simulink model "ProjectBosch"  (R2024b)
settings: Solver=FixedStepAuto  StartTime=0.0  StopTime=16000  FixedStep=1  RelTol=1e-3
libraries: simulink x5, embmathops x2
settings Model: Creator=user  LastModifiedBy=user

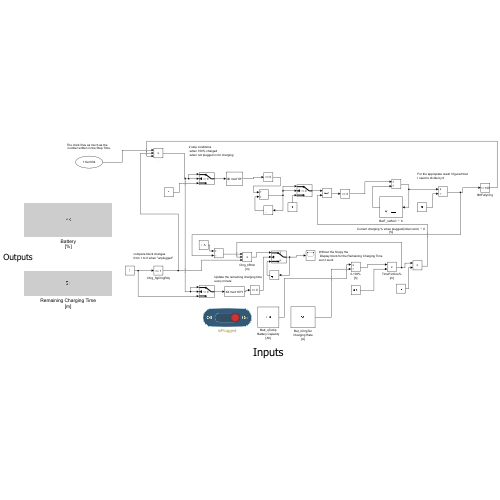
[thumbnail: Simulink's stored preview of the top-level diagram]
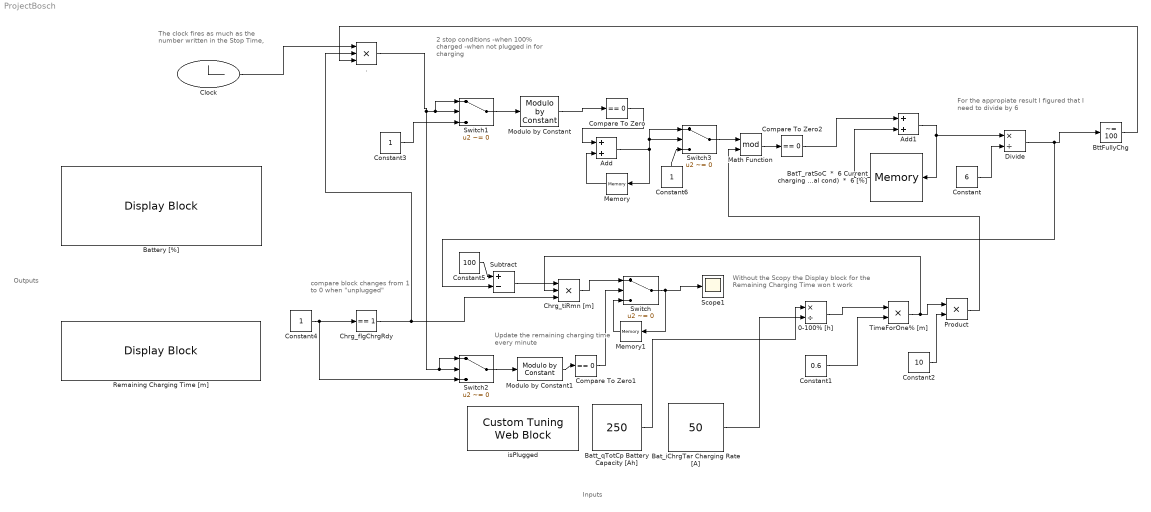
== system ProjectBosch ==
  note: Update the remaining charging time
      | every minute
  note: For the appropiate result I figured that
      | I need to divide by 6
  note: The clock fires as much as the
      |  number written in the Stop Time,
  note: Without the Scopy the
      |  Display block for the Remaining Charging Time
      | won t work
  note: compare block changes
      | from 1 to 0 when "unplugged"
  note: 2 stop conditions
      | -when 100% charged
      | -when not plugged in for charging
  note: Outputs
  note: Inputs
  . : Product  Inputs=3
  0-100% [h] : Product  Inputs=*/
  Add : Sum
  Add1 : Sum  OutDataTypeStr=uint32
  BatT_ratSoC  *  6 Current charging % when plugged(initial cond)  *  6 [%] : Memory
  Bat_iChrgTar Charging Rate [A] : Constant  Value=50
  Batt_qTotCp Battery Capacity [Ah] : Constant  Value=250
  Battery [%] : DisplayBlock  LabelPosition=Hide  Transparency=1
  "BttFullyChg " : simulink/Logic and Bit Operations/Compare To Constant  relop=~=  const=100  OutDataTypeStr=boolean
  Chrg_flgChrgRdy : simulink/Logic and Bit Operations/Compare To Constant  relop===  const=1  OutDataTypeStr=boolean
  Chrg_tiRmn [m] : Product  Inputs=3
  Clock : Clock
  Compare To Zero : simulink/Logic and Bit Operations/Compare To Zero  relop===  OutDataTypeStr=uint8
  Compare To Zero1 : simulink/Logic and Bit Operations/Compare To Zero  relop===  OutDataTypeStr=boolean
  Compare To Zero2 : simulink/Logic and Bit Operations/Compare To Zero  relop===  OutDataTypeStr=uint8
  Constant : Constant  Value=6
  Constant1 : Constant  Value=0.6
  Constant2 : Constant  Value=10
  Constant3 : Constant
  Constant4 : Constant
  Constant5 : Constant  Value=100
  Constant6 : Constant
  Divide : Product  Inputs=*/
  Math Function : Math  Operator=mod
  Memory : Memory
  Memory1 : Memory
  Modulo by Constant : embmathops/Modulo by Constant  Denominator=6  SimulateUsing=Code generation
      settings: LibrarySourceBlock=embeddedMathLib/Modulo by Constant
  Modulo by Constant1 : embmathops/Modulo by Constant  Denominator=60  SimulateUsing=Code generation
      settings: LibrarySourceBlock=embeddedMathLib/Modulo by Constant
  Product : Product
  Remaining Charging Time [m] : DisplayBlock  LabelPosition=Hide  Transparency=1
  Scope1 : Scope
  Subtract : Sum  Inputs=+-
  Switch{,1..3} (4 alike) : Switch  Criteria=u2 ~= 0  SaturateOnIntegerOverflow=off  InputSameDT=off
  TimeForOne% [m] : Product
  isPlugged : CustomTuningWebBlock  LabelPosition=Hide  ShowInitialText=on  Configuration="{\"components\":[{\"name\":\"CustomSwitchStateComponent\",\"settings\":{\"position\":[0,0,1,1],\"states\":[{\"HitRegion\":{\"position\":[0,0,0.5,1]},\"Image\":{\"position\":[0,0,1,1],\"size\":[1,1],\"src\":\"data:image\\/svg+xml;base64,PD94bWwgdmVyc2lvbj0iMS4wIiBlbmNvZGluZz0idXRmLTgiPz4NCjwhLS0gR2VuZXJhdG9yOiBBZG9iZSBJbGx1c3RyYXRvciAyNS4yLjEsIFNWRyBFeHBvcnQgUGx1Zy1JbiAuIFNWRyBWZXJzaW9uOiA2LjAwIEJ1aWxkIDApICAtLT4NCjxzdmcgdmVyc2lvbj0iMS4xIiB4bWxucz0iaHR0cDovL3d3dy53My5vcmcvMjAwMC9zdmciIHhtbG5zOnhsaW5rPSJodHRwOi8vd3d3LnczLm9yZy8xOTk5L3hsaW5rIiB4PSIwcHgiIHk9IjBweCINCgkgdmlld0JveD0iMCAwIDc2IDI5IiBzdHlsZT0iZW5hYmxlLWJhY2tncm91bmQ6bmV3 ...(+5404 chars)\",\"srcOrientation\":\"Right\"},\"Label\":{\"color\":[0.9882352941176471,0.9882352941176471,0.7725490196078432],\"icon\":{\"size\":[0,0],\"src\":[],\"srcOrientation\":\"Right\"},\"iconOffset\":0,\"iconPlacement\":\"left\",\"opacity\":1,\"position\":[0.5,0.14],\"show\":true,\"text\":{\"content\":\"Off\",\"font\":\"Helvetica\"}},\"Value\":0},{\"HitRegion\":{\"position\":[0,0.5,0.5,1]},\"Image\":{\"position\":[0,0,1,1],\"size\":[1,1],\"src\":\"data:image\\/svg+xml;base64,PD94bWwgdmVyc2lvbj0iMS4wIiBlbmNvZGluZz0idXRmLTgiPz4NCjwhLS0gR2VuZXJhdG9yOiBBZG9iZSBJbGx1c3RyYXRvciAyNS4yLjEsIFNWRyBFeHBvcnQgUGx1Zy1JbiAuIFNWRyBWZXJzaW9uOiA2LjAwIEJ1aWxkIDApICAtLT4NCjxzdmcgdmVyc2lvbj0iMS4xIiB4bWxucz0iaHR0cDovL3d3dy53My5vcmcvMjAwMC9zdmciIHhtbG5zOnhsaW5rPSJodHRwOi8vd3d3LnczLm9yZy8xOTk5L3hsaW5rIiB4PSIwcHgiIHk9IjBweCINCgkgdmlld0JveD0iMCAwIDc2IDI5IiBzdHlsZT0iZW5hYmxlLWJhY2tncm91bmQ6bmV3 ...(+5404 chars)\",\"srcOrientation\":\"Right\"},\"Label\":{\"color\":[0.9882352941176471,0.9882352941176471,0.7725490196078432],\"icon\":{\"size\":[0,0],\"src\":[],\"srcOrientation\":\"Right\"},\"iconOffset\":0,\"iconPlacement\":\"left\",\"opacity\":1,\"position\":[0.5,0.86],\"show\":true,\"text\":{\"content\":\"On\",\"font\":\"Helvetica\"}},\"Value\":1}]}},{\"name\":\"BackgroundImageComponent\",\"settings\":{\"image\":{\"size\":[140,55],\"src\":\"default\",\"srcOrientation\":\"Right\"},\"position\":[0,0,1,1],\"scaleMode\":\"0\"}},{\"name\":\"ForegroundImageComponent\",\"settings\":{\"image\":{\"size\":[0,0],\"src\":\"default\",\"srcOrientation\":[]},\"isForeground\":1,\"position\":[0,0,1,1],\"scaleMode\":\"0\"}}],\"settings\":{\"BindingType\":\"param\",\"backgroundColor\":[0,0,255,\"1\"],\"backgroundOffset\":0.14,\"fixedAspectRatio\":\"on\",\"foregroundColor\":[234,234,234],\"showBackgroundColor\":false,\"variant\":\"slider\",\"version\":\"R2024b\"},\"type\":\"Switch\"}"
  wires:
  Modulo by Constant/1 -> Compare To Zero/1
  Batt_qTotCp Battery Capacity [Ah]/1 -> 0-100% [h]/1
  Bat_iChrgTar Charging Rate [A]/1 -> 0-100% [h]/2
  Constant1/1 -> TimeForOne% [m]/2
  0-100% [h]/1 -> TimeForOne% [m]/1
  Compare To Zero/1 -> Add/1
  TimeForOne% [m]/1 -> Chrg_tiRmn [m]/2, Product/1
  Constant2/1 -> Product/2
  Product/1 -> Math Function/2
  Math Function/1 -> Compare To Zero2/1
  Add/1 -> Memory/1, Switch3/1, Switch3/2
  Memory/1 -> Add/2
  BatT_ratSoC  *  6 Current charging % when plugged(initial cond)  *  6 [%]/1 -> Add1/2
  Constant4/1 -> Switch2/3, Chrg_flgChrgRdy/1
  Constant5/1 -> Subtract/1
  Subtract/1 -> Chrg_tiRmn [m]/1
  Chrg_flgChrgRdy/1 -> ./2, Chrg_tiRmn [m]/3
  "BttFullyChg "/1 -> ./3
  Clock/1 -> ./1
  Modulo by Constant1/1 -> Compare To Zero1/1
  Compare To Zero2/1 -> Add1/1
  Constant/1 -> Divide/2
  Add1/1 -> Divide/1, BatT_ratSoC  *  6 Current charging % when plugged(initial cond)  *  6 [%]/1
  Divide/1 -> Subtract/2, "BttFullyChg "/1
  Compare To Zero1/1 -> Switch/2
  Chrg_tiRmn [m]/1 -> Switch/1
  Switch/1 -> Memory1/1, Scope1/1
  Memory1/1 -> Switch/3
  Switch1/1 -> Modulo by Constant/1
  Switch2/1 -> Modulo by Constant1/1
  Constant3/1 -> Switch1/3
  ./1 -> Switch2/1, Switch2/2, Switch1/1, Switch1/2
  Switch3/1 -> Math Function/1
  Constant6/1 -> Switch3/3
